simulink model "NM100A_MotVelCtrl"  (R2013b)
settings: Solver=FixedStepDiscrete  SolverMode=SingleTasking  StartTime=0.0  StopTime=1  FixedStep=0.002  RelTol=1e-3
values from neighbouring files (symbols this model uses):
  ARCHGLBPRM_2MILLISEC_SEC_F32 = DataDict.Constant    [NM100A_MotVelCtrl_DataDict.m]
  DERIVTVLPFILTICONLOWRLIM_SEC_F32 = DataDict.Constant    [NM100A_MotVelCtrl_DataDict.m]
  FALSE_CNT_LGC = DataDict.Constant    [NM100A_MotVelCtrl_DataDict.m]
  MOTVELTHDRAMPDWNCMPL_MOTRADPERSEC_F32 = DataDict.Constant    [NM100A_MotVelCtrl_DataDict.m]
  ONEMILLISEC_SEC_F32 = DataDict.Constant    [NM100A_MotVelCtrl_DataDict.m]
  TITHDRAMPDWNCMPL_CNT_U16 = DataDict.Constant    [NM100A_MotVelCtrl_DataDict.m]
  TRUE_CNT_LGC = DataDict.Constant    [NM100A_MotVelCtrl_DataDict.m]
  ZEROMOTVELTAR_MOTRADPERSEC_F32 = DataDict.Constant    [NM100A_MotVelCtrl_DataDict.m]
  ZEROTQCMD_MOTNWTMTR_F32 = DataDict.Constant    [NM100A_MotVelCtrl_DataDict.m]
libraries: NxtrLim x13, simulink x1, NxtrAbslt x1, NxtrMax x1
(part 1 of 4)
settings Model: Creator=DZVCQL  LastModifiedBy=DZVCQL
settings SolverCC: AutoInsertRateTranBlk=on  InsertRTBMode=Always
settings DataIOCC: LimitDataPoints=off  SaveFormat=Structure  ReturnWorkspaceOutputs=on
settings OptimizationCC: BlockReduction=off  InlineParams=on  ZeroExternalMemoryAtStartup=off  ZeroInternalMemoryAtStartup=off  OptimizeModelRefInitCode=on  LifeSpan=1
settings DebuggingCC: SignalInfNanChecking=error  SignalRangeChecking=warning  ReadBeforeWriteMsg=DisableAll  WriteAfterWriteMsg=DisableAll  WriteAfterReadMsg=DisableAll  UnderspecifiedInitializationDetection=Simplified  SolverPrmCheckMsg=error  InheritedTsInSrcMsg=error  DiscreteInheritContinuousMsg=error  SingleTaskRateTransMsg=error  TasksWithSamePriorityMsg=error  SigSpecEnsureSampleTimeMsg=error  CheckMatrixSingularityMsg=error  ParameterUnderflowMsg=error  ParameterPrecisionLossMsg=error  ParameterTunabilityLossMsg=error  FixptConstUnderflowMsg=warning  FixptConstOverflowMsg=warning  VectorMatrixConversionMsg=error  SignalLabelMismatchMsg=error  UnconnectedInputMsg=error  UnconnectedOutputMsg=error  UnconnectedLineMsg=error  SFcnCompatibilityMsg=error  UniqueDataStoreMsg=warning  BusObjectLabelMismatch=error  RootOutportRequireBusObject=error  AssertControl=DisableAll  ModelReferenceIOMsg=error  ModelReferenceVersionMismatchMessage=warning  ModelReferenceIOMismatchMessage=error  ModelReferenceCSMismatchMessage=warning  ModelReferenceDataLoggingMessage=error  StateNameClashWarn=warning  StrictBusMsg=ErrorOnBusTreatedAsVector  NonBusSignalsTreatedAsBus=error  SFUnexpectedBacktrackingDiag=error  SFInvalidInputDataAccessInChartInitDiag=error  SFNoUnconditionalDefaultTransitionDiag=error  SFTransitionOutsideNaturalParentDiag=error  SFUnconditionalTransitionShadowingDiag=error  SFUndirectedBroadcastEventsDiag=error
settings ModelReferenceCC: ModelReferenceNumInstancesAllowed=Single
settings RTWCC: SystemTargetFile=autosar.tlc  GenCodeOnly=on  TemplateMakefile=ert_default_tmf  Description=AUTOSAR  GenerateReport=on  ProcessScript=autosar_make_rtw_hook  LaunchReport=on
settings CodeAppCC: GenerateComments=off  IgnoreCustomStorageClasses=off  CustomSymbolStrType=$N$R$M  CustomSymbolStrBlkIO=$N$M  SimulinkBlockComments=off
settings STFCustomTargetCC: ParMdlRefBuildCompliant=on  CompOptLevelCompliant=on  IncludeMdlTerminateFcn=off  CombineOutputUpdateFcns=on  SuppressErrorStatus=on  ERTFirstTimeCompliant=on  ERTCustomFileBanners=on  SupportNonFinite=off  SupportComplex=off  SupportContinuousTime=off  SupportNonInlinedSFcns=off  MATLABClassNameForMDSCustomization=Simulink.SoftwareTarget.ERTCustomization  AutosarCompliant=on  GRTInterface=off  SystemTargetFile=autosar.tlc
settings ERTTargetCC: CodeReplacementLibrary=ANSI_C  ConcurrentExecutionCompliant=off  IncludeMdlTerminateFcn=off  SuppressErrorStatus=on  SupportNonFinite=off  SupportComplex=off  ModelStepFunctionPrototypeControlCompliant=off  CPPClassGenCompliant=off  AutosarCompliant=on  InlinedParameterPlacement=NonHierarchical  ERTCustomFileTemplate=example_file_process.tlc  EnableUserReplacementTypes=on

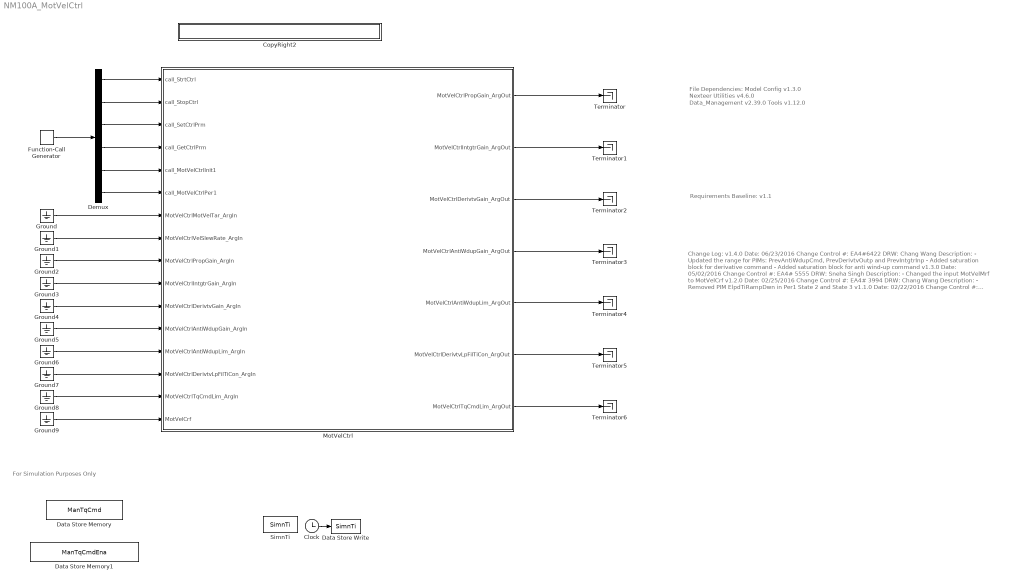
== system NM100A_MotVelCtrl ==
  note: Change Log:
      |
      | v1.4.0
      | Date: 06/23/2016
      | Change Control #: EA4#6422
      | DRW: Chang Wang
      | Description:
      | - Updated the range for PIMs: PrevAntiWdupCmd, PrevDerivtvOutp and PrevIntgtrInp
      | - Added saturation block for derivative command
      | - Added saturation block for anti wind-up command
      |
      | v1.3.0
      | Date: 05/02/2016
      | Change Control #: EA4# 5555
      | DRW: Sneha Singh
      | Description:
      | - Changed the input MotVelMrf to MotVelCrf
      |
      | v1.2.0
      | Date: 02/25/2016
      | Change Control #: EA4# 3994
      | DRW: Chang Wang
      | Description:
      | - Removed PIM ElpdTiRampDwn in Per1 State 2 and State 3
      |
      | v1.1.0
      | Date: 02/22/2016
      | Change Control #: EA4# 3954
      | DRW: Chang Wang
      | Description:
      | - Added client definition in data dictionary
      |
      | v1.0.0
      | Date: 02/09/2016
      | Change Control #: EA4# 2604
      | DRW: Chang Wang
      | Description:
      | - Initial Release
  note: Requirements Baseline: v1.1
  note: File Dependencies:
      |
      | Model Config v1.3.0
      | Nexteer Utilities v4.6.0
      | Data_Management v2.39.0
      | Tools v1.12.0
  note: For Simulation Purposes Only
  Clock : Clock
  CopyRight2 : Subsystem  Description=|  mask(Copyright Information){none=on}
      | Copyright info block.                                               
      |                                                                     
      | Place copyright information at the top of every subsystem in design.
      mask prompts: none "No parameters"
      mask help: Place copyright information at the top of every subsystem in design.
      mask Display:
      | NxtrConf = 'Nexteer Confidential';
      | 
      | sys = bdroot; %handle for the current model ("system")
      | first = get_param(sys,'Created');
      | if(isempty(first))
      |     first = datestr(now,'yyyy');
      | else
      |     first = first(end-3:end);  %year is last four digits
      | end
      | 
      | last = get_param(sys,'LastModifiedDate');
      | if isempty(last)
      |     last = datestr(now,'yyyy');
      | else
      |     last = last(end-3:end);
      | end
      | 
      | if strcmp(first,last)
      |     fprintf('%s -- Copyright %s Nexteer',NxtrConf,first)
      | else
      |     fprintf('%s -- %s%s- %s Nexteer',NxtrConf,char(169),first,last)
      | end
  Data Store Memory : DataStoreMemory  DataStoreName=ManTqCmd  ReadBeforeWriteMsg=warning  WriteAfterWriteMsg=warning  WriteAfterReadMsg=warning
  Data Store Memory1 : DataStoreMemory  DataStoreName=ManTqCmdEna  ReadBeforeWriteMsg=warning  WriteAfterWriteMsg=warning  WriteAfterReadMsg=warning
  Data Store Write : DataStoreWrite  DataStoreName=SimnTi
  Demux : Demux  Outputs=6
  Function-Call Generator : simulink/Ports & Subsystems/Function-Call Generator  sample_time=0.002  numberOfIterations=1
  Ground{,1..8} (9 alike) : Ground
  Ground9 : Ground  RequirementInfo="{}  %GIDa_4af75635_9092_474e_b30d_2604ca9b8832"
  MotVelCtrl : Subsystem
  SimnTi : DataStoreMemory  DataStoreName=SimnTi
  Terminator{,1..6} (7 alike) : Terminator
  wires:
  Demux/1 -> MotVelCtrl/1(call_StrtCtrl)
  Demux/2 -> MotVelCtrl/2(call_StopCtrl)
  Demux/3 -> MotVelCtrl/3(call_SetCtrlPrm)
  Demux/4 -> MotVelCtrl/4(call_GetCtrlPrm)
  Demux/5 -> MotVelCtrl/5(call_MotVelCtrlInit1)
  Demux/6 -> MotVelCtrl/6(call_MotVelCtrlPer1)
  Function-Call Generator/1 -> Demux/1
  Ground9/1 -> MotVelCtrl/16(MotVelCrf)
  Ground8/1 -> MotVelCtrl/15(MotVelCtrlTqCmdLim_ArgIn)
  Ground7/1 -> MotVelCtrl/14(MotVelCtrlDerivtvLpFilTiCon_ArgIn)
  Ground6/1 -> MotVelCtrl/13(MotVelCtrlAntiWdupLim_ArgIn)
  Ground5/1 -> MotVelCtrl/12(MotVelCtrlAntiWdupGain_ArgIn)
  Ground4/1 -> MotVelCtrl/11(MotVelCtrlDerivtvGain_ArgIn)
  Ground3/1 -> MotVelCtrl/10(MotVelCtrlIntgtrGain_ArgIn)
  Ground2/1 -> MotVelCtrl/9(MotVelCtrlPropGain_ArgIn)
  Ground1/1 -> MotVelCtrl/8(MotVelCtrlVelSlewRate_ArgIn)
  Ground/1 -> MotVelCtrl/7(MotVelCtrlMotVelTar_ArgIn)
  MotVelCtrl/1(MotVelCtrlPropGain_ArgOut) -> Terminator/1
  MotVelCtrl/2(MotVelCtrlIntgtrGain_ArgOut) -> Terminator1/1
  MotVelCtrl/3(MotVelCtrlDerivtvGain_ArgOut) -> Terminator2/1
  MotVelCtrl/4(MotVelCtrlAntiWdupGain_ArgOut) -> Terminator3/1
  MotVelCtrl/5(MotVelCtrlAntiWdupLim_ArgOut) -> Terminator4/1
  MotVelCtrl/6(MotVelCtrlDerivtvLpFilTiCon_ArgOut) -> Terminator5/1
  MotVelCtrl/7(MotVelCtrlTqCmdLim_ArgOut) -> Terminator6/1
  Clock/1 -> Data Store Write/1

== system NM100A_MotVelCtrl/CopyRight2 ==

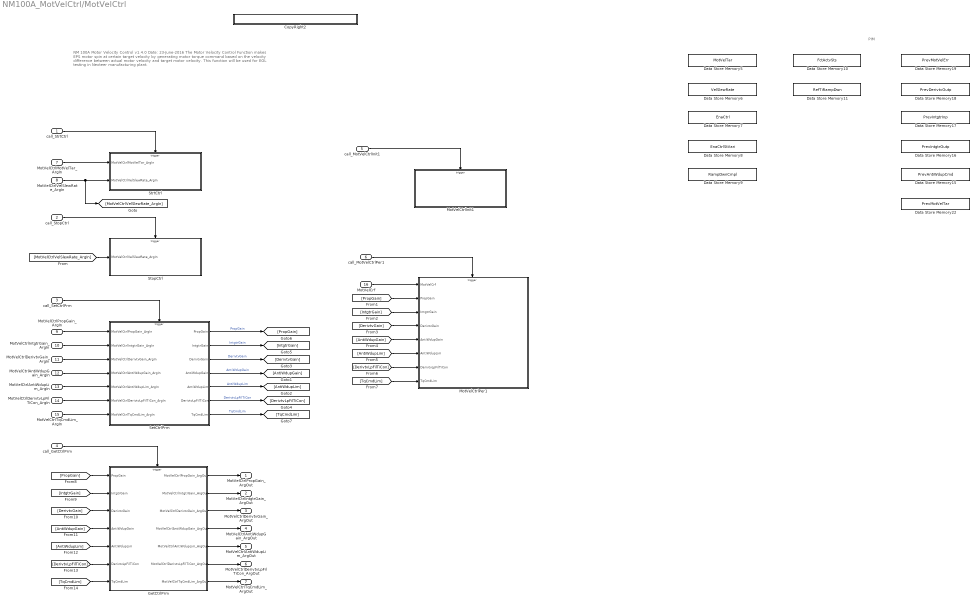
== system NM100A_MotVelCtrl/MotVelCtrl ==
  note: PIM
  note: NM 100A  Motor Velocity Control
      | v1.4.0      Date: 23-June-2016
      |
      | The Motor Velocity Control Function makes EPS motor spin at certain target velocity by generating motor torque command based on the
      | velocity difference between actual motor velocity and target motor velocity. This function will be used for EOL testing in Nexteer manufacturing
      | plant.
  call_StrtCtrl : Inport
  call_StopCtrl : Inport  Port=2
  call_SetCtrlPrm : Inport  Port=3
  call_GetCtrlPrm : Inport  Port=4
  call_MotVelCtrlInit1 : Inport  Port=5
  call_MotVelCtrlPer1 : Inport  Port=6
  MotVelCtrlMotVelTar_ArgIn : Inport  RequirementInfo="{'linktype_rmi_doors' '00010020 (/E-STEER Core/SubSystem Specifications/Manufacturing Service/NM100A_Motor Velocity Control Function Requirement)' '#NM100A_10' 'true' 'REQ:  NM100A_10' '' ; 'linktype_rmi_doors' '00010020 (/E-STEER Core/SubSystem Specifications/Manufacturing Service/NM100A_Motor Velocity Control Function Requirement)' '#NM100A_84' 'true' 'REQ:  NM100A_84' '' } %GIDa_b4e5afd2_56f5_46d2_aa0a_1f9c462eceac"  Port=7
  MotVelCtrlVelSlewRate_ArgIn : Inport  RequirementInfo="{'linktype_rmi_doors' '00010020 (/E-STEER Core/SubSystem Specifications/Manufacturing Service/NM100A_Motor Velocity Control Function Requirement)' '#NM100A_11' 'true' 'REQ:  NM100A_11' '' ; 'linktype_rmi_doors' '00010020 (/E-STEER Core/SubSystem Specifications/Manufacturing Service/NM100A_Motor Velocity Control Function Requirement)' '#NM100A_84' 'true' 'REQ:  NM100A_84' '' } %GIDa_6a002315_8dfa_4d7e_b831_7383949bc30b"  Port=8
  MotVelCtrlPropGain_ArgIn : Inport  RequirementInfo="{'linktype_rmi_doors' '00010020 (/E-STEER Core/SubSystem Specifications/Manufacturing Service/NM100A_Motor Velocity Control Function Requirement)' '#NM100A_13' 'true' 'REQ:  NM100A_13' '' ; 'linktype_rmi_doors' '00010020 (/E-STEER Core/SubSystem Specifications/Manufacturing Service/NM100A_Motor Velocity Control Function Requirement)' '#NM100A_85' 'true' 'REQ:  NM100A_85' '' } %GIDa_fa7a9d38_ec4e_42af_8ef7_a516fd31c72a"  Port=9
  MotVelCtrlIntgtrGain_ArgIn : Inport  RequirementInfo="{'linktype_rmi_doors' '00010020 (/E-STEER Core/SubSystem Specifications/Manufacturing Service/NM100A_Motor Velocity Control Function Requirement)' '#NM100A_13' 'true' 'REQ:  NM100A_13' '' ; 'linktype_rmi_doors' '00010020 (/E-STEER Core/SubSystem Specifications/Manufacturing Service/NM100A_Motor Velocity Control Function Requirement)' '#NM100A_85' 'true' 'REQ:  NM100A_85' '' } %GIDa_da1bc328_85e1_4524_82bb_c455a15a83f5"  Port=10
  MotVelCtrlDerivtvGain_ArgIn : Inport  RequirementInfo="{'linktype_rmi_doors' '00010020 (/E-STEER Core/SubSystem Specifications/Manufacturing Service/NM100A_Motor Velocity Control Function Requirement)' '#NM100A_13' 'true' 'REQ:  NM100A_13' '' ; 'linktype_rmi_doors' '00010020 (/E-STEER Core/SubSystem Specifications/Manufacturing Service/NM100A_Motor Velocity Control Function Requirement)' '#NM100A_85' 'true' 'REQ:  NM100A_85' '' } %GIDa_c5db38f5_dbd5_422b_8505_a0e67da4c1c3"  Port=11
  MotVelCtrlAntiWdupGain_ArgIn : Inport  RequirementInfo="{'linktype_rmi_doors' '00010020 (/E-STEER Core/SubSystem Specifications/Manufacturing Service/NM100A_Motor Velocity Control Function Requirement)' '#NM100A_14' 'true' 'REQ:  NM100A_14' '' ; 'linktype_rmi_doors' '00010020 (/E-STEER Core/SubSystem Specifications/Manufacturing Service/NM100A_Motor Velocity Control Function Requirement)' '#NM100A_85' 'true' 'REQ:  NM100A_85' '' } %GIDa_dd319c0c_aa78_494d_974e_a4fd1e8fae44"  Port=12
  MotVelCtrlAntiWdupLim_ArgIn : Inport  RequirementInfo="{'linktype_rmi_doors' '00010020 (/E-STEER Core/SubSystem Specifications/Manufacturing Service/NM100A_Motor Velocity Control Function Requirement)' '#NM100A_14' 'true' 'REQ:  NM100A_14' '' ; 'linktype_rmi_doors' '00010020 (/E-STEER Core/SubSystem Specifications/Manufacturing Service/NM100A_Motor Velocity Control Function Requirement)' '#NM100A_85' 'true' 'REQ:  NM100A_85' '' } %GIDa_0e3b6542_1c91_470d_a92d_ce3c261459b8"  Port=13
  MotVelCtrlDerivtvLpFilTiCon_ArgIn : Inport  RequirementInfo="{'linktype_rmi_doors' '00010020 (/E-STEER Core/SubSystem Specifications/Manufacturing Service/NM100A_Motor Velocity Control Function Requirement)' '#NM100A_15' 'true' 'REQ:  NM100A_15' '' ; 'linktype_rmi_doors' '00010020 (/E-STEER Core/SubSystem Specifications/Manufacturing Service/NM100A_Motor Velocity Control Function Requirement)' '#NM100A_85' 'true' 'REQ:  NM100A_85' '' } %GIDa_cfe3ce5c_c322_4f86_b6db_5a668332a15c"  Port=14
  MotVelCtrlTqCmdLim_ArgIn : Inport  RequirementInfo="{'linktype_rmi_doors' '00010020 (/E-STEER Core/SubSystem Specifications/Manufacturing Service/NM100A_Motor Velocity Control Function Requirement)' '#NM100A_16' 'true' 'REQ:  NM100A_16' '' ; 'linktype_rmi_doors' '00010020 (/E-STEER Core/SubSystem Specifications/Manufacturing Service/NM100A_Motor Velocity Control Function Requirement)' '#NM100A_85' 'true' 'REQ:  NM100A_85' '' } %GIDa_2c1dfec7_b849_4afb_8c15_4e0ef5eb7c29"  Port=15
  MotVelCrf : Inport  RequirementInfo="{'linktype_rmi_doors' '00010020 (/E-STEER Core/SubSystem Specifications/Manufacturing Service/NM100A_Motor Velocity Control Function Requirement)' '#NM100A_9' 'true' 'REQ:  NM100A_9' '' } %GIDa_78fb18dd_9313_48f8_8b5a_3efff0ddc69b"  Port=16
  CopyRight2 : Subsystem  Description=|  mask(Copyright Information){none=on}
      | Copyright info block.                                               
      |                                                                     
      | Place copyright information at the top of every subsystem in design.
      mask prompts: none "No parameters"
      mask help: Place copyright information at the top of every subsystem in design.
      mask Display:
      | NxtrConf = 'Nexteer Confidential';
      | 
      | sys = bdroot; %handle for the current model ("system")
      | first = get_param(sys,'Created');
      | if(isempty(first))
      |     first = datestr(now,'yyyy');
      | else
      |     first = first(end-3:end);  %year is last four digits
      | end
      | 
      | last = get_param(sys,'LastModifiedDate');
      | if isempty(last)
      |     last = datestr(now,'yyyy');
      | else
      |     last = last(end-3:end);
      | end
      | 
      | if strcmp(first,last)
      |     fprintf('%s -- Copyright %s Nexteer',NxtrConf,first)
      | else
      |     fprintf('%s -- %s%s- %s Nexteer',NxtrConf,char(169),first,last)
      | end
  Data Store Memory10 : DataStoreMemory  DataStoreName=FctActvSts  ReadBeforeWriteMsg=warning  WriteAfterWriteMsg=warning  WriteAfterReadMsg=warning  StateMustResolveToSignalObject=on
  Data Store Memory11 : DataStoreMemory  DataStoreName=RefTiRampDwn  ReadBeforeWriteMsg=warning  WriteAfterWriteMsg=warning  WriteAfterReadMsg=warning  StateMustResolveToSignalObject=on
  Data Store Memory15 : DataStoreMemory  DataStoreName=PrevAntiWdupCmd  ReadBeforeWriteMsg=warning  WriteAfterWriteMsg=warning  WriteAfterReadMsg=warning  StateMustResolveToSignalObject=on
  Data Store Memory16 : DataStoreMemory  DataStoreName=PrevIntgtrOutp  ReadBeforeWriteMsg=warning  WriteAfterWriteMsg=warning  WriteAfterReadMsg=warning  StateMustResolveToSignalObject=on
  Data Store Memory17 : DataStoreMemory  DataStoreName=PrevIntgtrInp  ReadBeforeWriteMsg=warning  WriteAfterWriteMsg=warning  WriteAfterReadMsg=warning  StateMustResolveToSignalObject=on
  Data Store Memory18 : DataStoreMemory  DataStoreName=PrevDerivtvOutp  ReadBeforeWriteMsg=warning  WriteAfterWriteMsg=warning  WriteAfterReadMsg=warning  StateMustResolveToSignalObject=on
  Data Store Memory19 : DataStoreMemory  DataStoreName=PrevMotVelErr  ReadBeforeWriteMsg=warning  WriteAfterWriteMsg=warning  WriteAfterReadMsg=warning  StateMustResolveToSignalObject=on
  Data Store Memory22 : DataStoreMemory  DataStoreName=PrevMotVelTar  ReadBeforeWriteMsg=warning  WriteAfterWriteMsg=warning  WriteAfterReadMsg=warning  StateMustResolveToSignalObject=on
  Data Store Memory5 : DataStoreMemory  DataStoreName=MotVelTar  ReadBeforeWriteMsg=warning  WriteAfterWriteMsg=warning  WriteAfterReadMsg=warning  StateMustResolveToSignalObject=on
  Data Store Memory6 : DataStoreMemory  DataStoreName=VelSlewRate  ReadBeforeWriteMsg=warning  WriteAfterWriteMsg=warning  WriteAfterReadMsg=warning  StateMustResolveToSignalObject=on
  Data Store Memory7 : DataStoreMemory  DataStoreName=EnaCtrl  ReadBeforeWriteMsg=warning  WriteAfterWriteMsg=warning  WriteAfterReadMsg=warning  StateMustResolveToSignalObject=on
  Data Store Memory8 : DataStoreMemory  DataStoreName=EnaCtrlStVari  ReadBeforeWriteMsg=warning  WriteAfterWriteMsg=warning  WriteAfterReadMsg=warning  StateMustResolveToSignalObject=on
  Data Store Memory9 : DataStoreMemory  DataStoreName=RampDwnCmpl  ReadBeforeWriteMsg=warning  WriteAfterWriteMsg=warning  WriteAfterReadMsg=warning  StateMustResolveToSignalObject=on
  GetCtrlPrm : Subsystem  TreatAsAtomicUnit=on
  MotVelCtrlInit1 : Subsystem  TreatAsAtomicUnit=on
  MotVelCtrlPer1 : Subsystem  TreatAsAtomicUnit=on
  SetCtrlPrm : Subsystem  TreatAsAtomicUnit=on
  StopCtrl : Subsystem  TreatAsAtomicUnit=on
  StrtCtrl : Subsystem  TreatAsAtomicUnit=on
  MotVelCtrlPropGain_ArgOut : Outport  RequirementInfo="{'linktype_rmi_doors' '00010020 (/E-STEER Core/SubSystem Specifications/Manufacturing Service/NM100A_Motor Velocity Control Function Requirement)' '#NM100A_105' 'true' 'REQ:  NM100A_105' '' ; 'linktype_rmi_doors' '00010020 (/E-STEER Core/SubSystem Specifications/Manufacturing Service/NM100A_Motor Velocity Control Function Requirement)' '#NM100A_86' 'true' 'REQ:  NM100A_86' '' } %GIDa_fbcf257f_3a7e_4784_95d9_7f44ee96f49e"
  MotVelCtrlIntgtrGain_ArgOut : Outport  RequirementInfo="{'linktype_rmi_doors' '00010020 (/E-STEER Core/SubSystem Specifications/Manufacturing Service/NM100A_Motor Velocity Control Function Requirement)' '#NM100A_105' 'true' 'REQ:  NM100A_105' '' ; 'linktype_rmi_doors' '00010020 (/E-STEER Core/SubSystem Specifications/Manufacturing Service/NM100A_Motor Velocity Control Function Requirement)' '#NM100A_86' 'true' 'REQ:  NM100A_86' '' } %GIDa_a30212a1_db40_493f_99ad_7cd60670be6b"  Port=2
  MotVelCtrlDerivtvGain_ArgOut : Outport  RequirementInfo="{'linktype_rmi_doors' '00010020 (/E-STEER Core/SubSystem Specifications/Manufacturing Service/NM100A_Motor Velocity Control Function Requirement)' '#NM100A_105' 'true' 'REQ:  NM100A_105' '' ; 'linktype_rmi_doors' '00010020 (/E-STEER Core/SubSystem Specifications/Manufacturing Service/NM100A_Motor Velocity Control Function Requirement)' '#NM100A_86' 'true' 'REQ:  NM100A_86' '' } %GIDa_d511169f_960f_4b26_aa3f_53333eb486bd"  Port=3
  MotVelCtrlAntiWdupGain_ArgOut : Outport  RequirementInfo="{'linktype_rmi_doors' '00010020 (/E-STEER Core/SubSystem Specifications/Manufacturing Service/NM100A_Motor Velocity Control Function Requirement)' '#NM100A_107' 'true' 'REQ:  NM100A_107' '' ; 'linktype_rmi_doors' '00010020 (/E-STEER Core/SubSystem Specifications/Manufacturing Service/NM100A_Motor Velocity Control Function Requirement)' '#NM100A_86' 'true' 'REQ:  NM100A_86' '' } %GIDa_da526535_3849_41c7_869e_59d948236c9d"  Port=4
  MotVelCtrlAntiWdupLim_ArgOut : Outport  RequirementInfo="{'linktype_rmi_doors' '00010020 (/E-STEER Core/SubSystem Specifications/Manufacturing Service/NM100A_Motor Velocity Control Function Requirement)' '#NM100A_107' 'true' 'REQ:  NM100A_107' '' ; 'linktype_rmi_doors' '00010020 (/E-STEER Core/SubSystem Specifications/Manufacturing Service/NM100A_Motor Velocity Control Function Requirement)' '#NM100A_86' 'true' 'REQ:  NM100A_86' '' } %GIDa_a2928b64_1a88_4f0b_886a_22a0a7f92bff"  Port=5
  MotVelCtrlDerivtvLpFilTiCon_ArgOut : Outport  RequirementInfo="{'linktype_rmi_doors' '00010020 (/E-STEER Core/SubSystem Specifications/Manufacturing Service/NM100A_Motor Velocity Control Function Requirement)' '#NM100A_108' 'true' 'REQ:  NM100A_108' '' ; 'linktype_rmi_doors' '00010020 (/E-STEER Core/SubSystem Specifications/Manufacturing Service/NM100A_Motor Velocity Control Function Requirement)' '#NM100A_86' 'true' 'REQ:  NM100A_86' '' } %GIDa_e78ab4ff_8646_49da_9642_5dd7cce604f1"  Port=6
  MotVelCtrlTqCmdLim_ArgOut : Outport  RequirementInfo="{'linktype_rmi_doors' '00010020 (/E-STEER Core/SubSystem Specifications/Manufacturing Service/NM100A_Motor Velocity Control Function Requirement)' '#NM100A_109' 'true' 'REQ:  NM100A_109' '' ; 'linktype_rmi_doors' '00010020 (/E-STEER Core/SubSystem Specifications/Manufacturing Service/NM100A_Motor Velocity Control Function Requirement)' '#NM100A_86' 'true' 'REQ:  NM100A_86' '' } %GIDa_332bdf64_fdb5_47d8_90a4_34844676e793"  Port=7
  wires:
  call_StrtCtrl/1 -> StrtCtrl/Trigger
  MotVelCtrlMotVelTar_ArgIn/1 -> StrtCtrl/1(MotVelCtrlMotVelTar_ArgIn)
  MotVelCtrlVelSlewRate_ArgIn/1 -> [MotVelCtrlVelSlewRate_ArgIn], StrtCtrl/2(MotVelCtrlVelSlewRate_ArgIn)
  call_StopCtrl/1 -> StopCtrl/Trigger
  call_SetCtrlPrm/1 -> SetCtrlPrm/Trigger
  MotVelCtrlPropGain_ArgIn/1 -> SetCtrlPrm/1(MotVelCtrlPropGain_ArgIn)
  MotVelCtrlIntgtrGain_ArgIn/1 -> SetCtrlPrm/2(MotVelCtrlIntgtrGain_ArgIn)
  MotVelCtrlDerivtvGain_ArgIn/1 -> SetCtrlPrm/3(MotVelCtrlDerivtvGain_ArgIn)
  call_GetCtrlPrm/1 -> GetCtrlPrm/Trigger
  MotVelCtrlAntiWdupGain_ArgIn/1 -> SetCtrlPrm/4(MotVelCtrlAntiWdupGain_ArgIn)
  MotVelCtrlAntiWdupLim_ArgIn/1 -> SetCtrlPrm/5(MotVelCtrlAntiWdupLim_ArgIn)
  MotVelCtrlDerivtvLpFilTiCon_ArgIn/1 -> SetCtrlPrm/6(MotVelCtrlDerivtvLpFilTiCon_ArgIn)
  MotVelCtrlTqCmdLim_ArgIn/1 -> SetCtrlPrm/7(MotVelCtrlTqCmdLim_ArgIn)
  GetCtrlPrm/1(MotVelCtrlPropGain_ArgOut) -> MotVelCtrlPropGain_ArgOut/1
  GetCtrlPrm/2(MotVelCtrlIntgtrGain_ArgOut) -> MotVelCtrlIntgtrGain_ArgOut/1
  GetCtrlPrm/7(MotVelCtrlTqCmdLim_ArgOut) -> MotVelCtrlTqCmdLim_ArgOut/1
  GetCtrlPrm/6(MotVelCtrlDerivtvLpFilTiCon_ArgOut) -> MotVelCtrlDerivtvLpFilTiCon_ArgOut/1
  GetCtrlPrm/5(MotVelCtrlAntiWdupLim_ArgOut) -> MotVelCtrlAntiWdupLim_ArgOut/1
  GetCtrlPrm/4(MotVelCtrlAntiWdupGain_ArgOut) -> MotVelCtrlAntiWdupGain_ArgOut/1
  GetCtrlPrm/3(MotVelCtrlDerivtvGain_ArgOut) -> MotVelCtrlDerivtvGain_ArgOut/1
  [MotVelCtrlVelSlewRate_ArgIn] -> StopCtrl/1(MotVelCtrlVelSlewRate_ArgIn)
  call_MotVelCtrlPer1/1 -> MotVelCtrlPer1/Trigger
  MotVelCrf/1 -> MotVelCtrlPer1/1(MotVelCrf)
  call_MotVelCtrlInit1/1 -> MotVelCtrlInit1/Trigger
  SetCtrlPrm/1(PropGain) -> [PropGain]  "PropGain"
  SetCtrlPrm/2(IntgtrGain) -> [IntgtrGain]  "IntgtrGain"
  SetCtrlPrm/3(DerivtvGain) -> [DerivtvGain]  "DerivtvGain"
  SetCtrlPrm/4(AntiWdupGain) -> [AntiWdupGain]  "AntiWdupGain"
  SetCtrlPrm/5(AntiWdupLim) -> [AntiWdupLim]  "AntiWdupLim"
  SetCtrlPrm/6(DerivtvLpFilTiCon) -> [DerivtvLpFilTiCon]  "DerivtvLpFilTiCon"
  SetCtrlPrm/7(TqCmdLim) -> [TqCmdLim]  "TqCmdLim"
  [PropGain] -> GetCtrlPrm/1(PropGain)
  [IntgtrGain] -> GetCtrlPrm/2(IntgtrGain)
  [DerivtvGain] -> GetCtrlPrm/3(DerivtvGain)
  [AntiWdupGain] -> GetCtrlPrm/4(AntiWdupGain)
  [AntiWdupLim] -> GetCtrlPrm/5(AntiWdupLim)
  [DerivtvLpFilTiCon] -> GetCtrlPrm/6(DerivtvLpFilTiCon)
  [TqCmdLim] -> GetCtrlPrm/7(TqCmdLim)
  [PropGain] -> MotVelCtrlPer1/2(PropGain)
  [IntgtrGain] -> MotVelCtrlPer1/3(IntgtrGain)
  [DerivtvGain] -> MotVelCtrlPer1/4(DerivtvGain)
  [AntiWdupGain] -> MotVelCtrlPer1/5(AntiWdupGain)
  [AntiWdupLim] -> MotVelCtrlPer1/6(AntiWdupLim)
  [DerivtvLpFilTiCon] -> MotVelCtrlPer1/7(DerivtvLpFilTiCon)
  [TqCmdLim] -> MotVelCtrlPer1/8(TqCmdLim)

== system NM100A_MotVelCtrl/MotVelCtrl/CopyRight2 ==

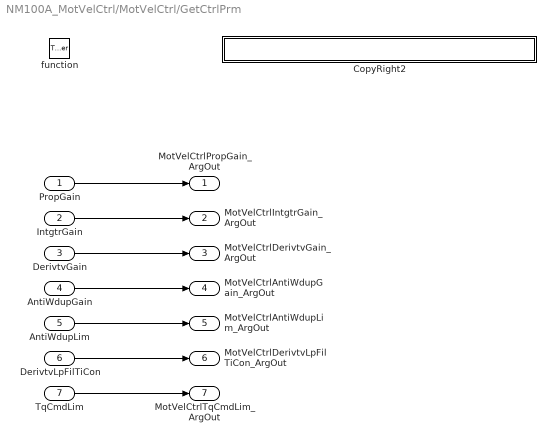
== system NM100A_MotVelCtrl/MotVelCtrl/GetCtrlPrm ==
  PropGain : Inport
  IntgtrGain : Inport  Port=2
  DerivtvGain : Inport  Port=3
  AntiWdupGain : Inport  Port=4
  AntiWdupLim : Inport  Port=5
  DerivtvLpFilTiCon : Inport  Port=6
  TqCmdLim : Inport  Port=7
  function : TriggerPort  TriggerType=function-call
  CopyRight2 : Subsystem  Description=|  mask(Copyright Information){none=on}
      | Copyright info block.                                               
      |                                                                     
      | Place copyright information at the top of every subsystem in design.
      mask prompts: none "No parameters"
      mask help: Place copyright information at the top of every subsystem in design.
      mask Display:
      | NxtrConf = 'Nexteer Confidential';
      | 
      | sys = bdroot; %handle for the current model ("system")
      | first = get_param(sys,'Created');
      | if(isempty(first))
      |     first = datestr(now,'yyyy');
      | else
      |     first = first(end-3:end);  %year is last four digits
      | end
      | 
      | last = get_param(sys,'LastModifiedDate');
      | if isempty(last)
      |     last = datestr(now,'yyyy');
      | else
      |     last = last(end-3:end);
      | end
      | 
      | if strcmp(first,last)
      |     fprintf('%s -- Copyright %s Nexteer',NxtrConf,first)
      | else
      |     fprintf('%s -- %s%s- %s Nexteer',NxtrConf,char(169),first,last)
      | end
  MotVelCtrlPropGain_ArgOut : Outport
  MotVelCtrlIntgtrGain_ArgOut : Outport  Port=2
  MotVelCtrlDerivtvGain_ArgOut : Outport  Port=3
  MotVelCtrlAntiWdupGain_ArgOut : Outport  Port=4
  MotVelCtrlAntiWdupLim_ArgOut : Outport  Port=5
  MotVelCtrlDerivtvLpFilTiCon_ArgOut : Outport  Port=6
  MotVelCtrlTqCmdLim_ArgOut : Outport  Port=7
  wires:
  TqCmdLim/1 -> MotVelCtrlTqCmdLim_ArgOut/1
  DerivtvLpFilTiCon/1 -> MotVelCtrlDerivtvLpFilTiCon_ArgOut/1
  AntiWdupLim/1 -> MotVelCtrlAntiWdupLim_ArgOut/1
  AntiWdupGain/1 -> MotVelCtrlAntiWdupGain_ArgOut/1
  DerivtvGain/1 -> MotVelCtrlDerivtvGain_ArgOut/1
  IntgtrGain/1 -> MotVelCtrlIntgtrGain_ArgOut/1
  PropGain/1 -> MotVelCtrlPropGain_ArgOut/1

== system NM100A_MotVelCtrl/MotVelCtrl/MotVelCtrlInit1 ==
  function : TriggerPort  TriggerType=function-call
  Constant : Constant  Value=FALSE_CNT_LGC
  Constant1 : Constant  Value=FALSE_CNT_LGC
  Constant2 : Constant  Value=TRUE_CNT_LGC
  Constant3 : Constant  Value=FALSE_CNT_LGC
  CopyRight2 : Subsystem  Description=|  mask(Copyright Information){none=on}
      | Copyright info block.                                               
      |                                                                     
      | Place copyright information at the top of every subsystem in design.
      mask prompts: none "No parameters"
      mask help: Place copyright information at the top of every subsystem in design.
      mask Display:
      | NxtrConf = 'Nexteer Confidential';
      | 
      | sys = bdroot; %handle for the current model ("system")
      | first = get_param(sys,'Created');
      | if(isempty(first))
      |     first = datestr(now,'yyyy');
      | else
      |     first = first(end-3:end);  %year is last four digits
      | end
      | 
      | last = get_param(sys,'LastModifiedDate');
      | if isempty(last)
      |     last = datestr(now,'yyyy');
      | else
      |     last = last(end-3:end);
      | end
      | 
      | if strcmp(first,last)
      |     fprintf('%s -- Copyright %s Nexteer',NxtrConf,first)
      | else
      |     fprintf('%s -- %s%s- %s Nexteer',NxtrConf,char(169),first,last)
      | end
  Data Store Write : DataStoreWrite  DataStoreName=EnaCtrl
  Data Store Write1 : DataStoreWrite  DataStoreName=EnaCtrlStVari
  Data Store Write2 : DataStoreWrite  DataStoreName=RampDwnCmpl
  Data Store Write3 : DataStoreWrite  DataStoreName=FctActvSts
  wires:
  Constant/1 -> Data Store Write/1
  Constant1/1 -> Data Store Write1/1
  Constant2/1 -> Data Store Write2/1
  Constant3/1 -> Data Store Write3/1

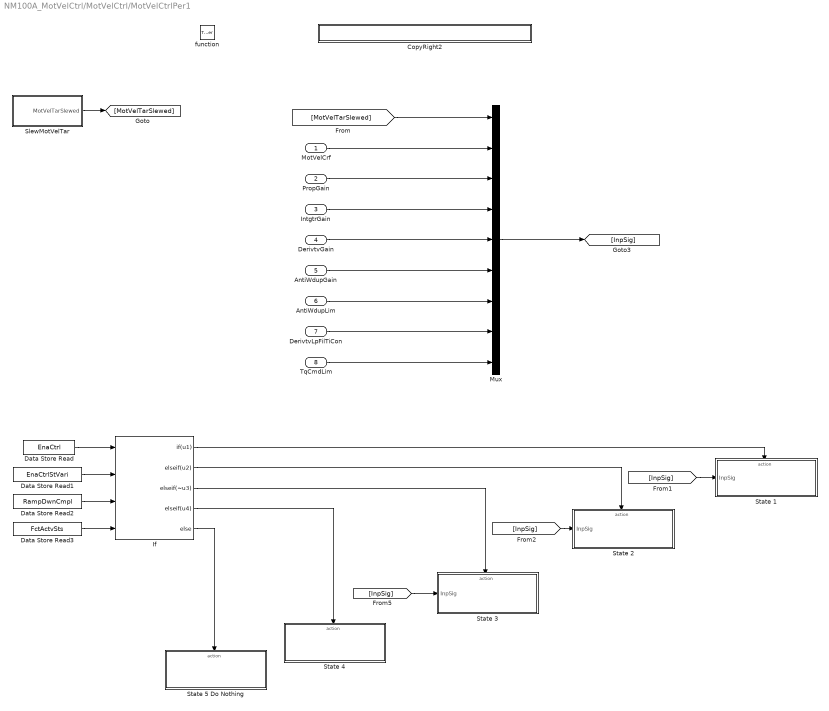
== system NM100A_MotVelCtrl/MotVelCtrl/MotVelCtrlPer1 ==
  MotVelCrf : Inport  RequirementInfo={} %GIDa_f6b199e4_d761_4852_9315_a0e807dc48bc
  PropGain : Inport  Port=2
  IntgtrGain : Inport  Port=3
  DerivtvGain : Inport  Port=4
  AntiWdupGain : Inport  Port=5
  AntiWdupLim : Inport  Port=6
  DerivtvLpFilTiCon : Inport  Port=7
  TqCmdLim : Inport  Port=8
  function : TriggerPort  TriggerType=function-call
  CopyRight2 : Subsystem  Description=|  mask(Copyright Information){none=on}
      | Copyright info block.                                               
      |                                                                     
      | Place copyright information at the top of every subsystem in design.
      mask prompts: none "No parameters"
      mask help: Place copyright information at the top of every subsystem in design.
      mask Display:
      | NxtrConf = 'Nexteer Confidential';
      | 
      | sys = bdroot; %handle for the current model ("system")
      | first = get_param(sys,'Created');
      | if(isempty(first))
      |     first = datestr(now,'yyyy');
      | else
      |     first = first(end-3:end);  %year is last four digits
      | end
      | 
      | last = get_param(sys,'LastModifiedDate');
      | if isempty(last)
      |     last = datestr(now,'yyyy');
      | else
      |     last = last(end-3:end);
      | end
      | 
      | if strcmp(first,last)
      |     fprintf('%s -- Copyright %s Nexteer',NxtrConf,first)
      | else
      |     fprintf('%s -- %s%s- %s Nexteer',NxtrConf,char(169),first,last)
      | end
  Data Store Read : DataStoreRead  RequirementInfo="{'linktype_rmi_doors' '00010020 (/E-STEER Core/SubSystem Specifications/Manufacturing Service/NM100A_Motor Velocity Control Function Requirement)' '#NM100A_48' 'true' 'REQ:  NM100A_48' '' ; 'linktype_rmi_doors' '00010020 (/E-STEER Core/SubSystem Specifications/Manufacturing Service/NM100A_Motor Velocity Control Function Requirement)' '#NM100A_49' 'true' 'REQ:  NM100A_49' '' ; 'linktype_rmi_doors' '00010020 (/E-STEER Core/SubSystem Specifications/Manufacturing Service/NM100A_Motor Velocity Control Function Requirement)' '#NM100A_51' 'true' 'REQ:  NM100A_51' '' ; 'linktype_rmi_doors' '00010020 (/E-STEER Core/SubSystem Specifications/Manufacturing Service/NM100A_Motor Velocity Control Function Requirement)' '#NM100A_103' 'true' 'REQ:  NM100A_103' '' } %GIDa_43add5bf_a7cd_4f8a_9e70_c6a4259d43f2"  DataStoreName=EnaCtrl
  Data Store Read1 : DataStoreRead  RequirementInfo="{'linktype_rmi_doors' '00010020 (/E-STEER Core/SubSystem Specifications/Manufacturing Service/NM100A_Motor Velocity Control Function Requirement)' '#NM100A_49' 'true' 'REQ:  NM100A_49' '' ; 'linktype_rmi_doors' '00010020 (/E-STEER Core/SubSystem Specifications/Manufacturing Service/NM100A_Motor Velocity Control Function Requirement)' '#NM100A_51' 'true' 'REQ:  NM100A_51' '' ; 'linktype_rmi_doors' '00010020 (/E-STEER Core/SubSystem Specifications/Manufacturing Service/NM100A_Motor Velocity Control Function Requirement)' '#NM100A_103' 'true' 'REQ:  NM100A_103' '' } %GIDa_56e92a46_fc14_4f42_a1bf_376f15bd98ae"  DataStoreName=EnaCtrlStVari
  Data Store Read2 : DataStoreRead  RequirementInfo="{'linktype_rmi_doors' '00010020 (/E-STEER Core/SubSystem Specifications/Manufacturing Service/NM100A_Motor Velocity Control Function Requirement)' '#NM100A_51' 'true' 'REQ:  NM100A_51' '' ; 'linktype_rmi_doors' '00010020 (/E-STEER Core/SubSystem Specifications/Manufacturing Service/NM100A_Motor Velocity Control Function Requirement)' '#NM100A_103' 'true' 'REQ:  NM100A_103' '' } %GIDa_d16d24dc_3caf_4308_b6b9_14741c0660fb"  DataStoreName=RampDwnCmpl
  Data Store Read3 : DataStoreRead  RequirementInfo="{'linktype_rmi_doors' '00010020 (/E-STEER Core/SubSystem Specifications/Manufacturing Service/NM100A_Motor Velocity Control Function Requirement)' '#NM100A_103' 'true' 'REQ:  NM100A_103' '' } %GIDa_dc81bd03_ef6f_4e75_8bbb_45c102c73405"  DataStoreName=FctActvSts
  If : If  RequirementInfo="{'linktype_rmi_doors' '00010020 (/E-STEER Core/SubSystem Specifications/Manufacturing Service/NM100A_Motor Velocity Control Function Requirement)' '#NM100A_48' 'true' 'REQ:  NM100A_48' '' ; 'linktype_rmi_doors' '00010020 (/E-STEER Core/SubSystem Specifications/Manufacturing Service/NM100A_Motor Velocity Control Function Requirement)' '#NM100A_49' 'true' 'REQ:  NM100A_49' '' ; 'linktype_rmi_doors' '00010020 (/E-STEER Core/SubSystem Specifications/Manufacturing Service/NM100A_Motor Velocity Control Function Requirement)' '#NM100A_51' 'true' 'REQ:  NM100A_51' '' ; 'linktype_rmi_doors' '00010020 (/E-STEER Core/SubSystem Specifications/Manufacturing Service/NM100A_Motor Velocity Control Function Requirement)' '#NM100A_103' 'true' 'REQ:  NM100A_103' '' ; 'linktype_rmi_doors' '00010020 (/E-STEER Core/SubSystem Specifications/Manufacturing Service/NM100A_Motor Velocity Control Function Requirement)' '#NM100A_130' 'true' 'REQ:  NM100A_130' '' } %GIDa_214f0c17_e692_4fb0_8ef6_fb165d366702"  NumInputs=4  IfExpression=u1  ElseIfExpressions=u2, ~u3, u4
  Mux : Mux  Inputs=9
  SlewMotVelTar : Subsystem
  State 1 : Subsystem  RequirementInfo={} %GIDa_8c6205ae_5932_444d_8028_d45b85e6549f  TreatAsAtomicUnit=on
  State 2 : Subsystem  RequirementInfo={} %GIDa_facb0b74_d7f2_406b_9dad_c80376ac3792  TreatAsAtomicUnit=on
  State 3 : Subsystem  TreatAsAtomicUnit=on
  State 4 : Subsystem  TreatAsAtomicUnit=on
  State 5 Do Nothing : Subsystem  RequirementInfo="{'linktype_rmi_doors' '00010020 (/E-STEER Core/SubSystem Specifications/Manufacturing Service/NM100A_Motor Velocity Control Function Requirement)' '#NM100A_130' 'true' 'REQ:  NM100A_130' '' } %GIDa_98eb7df3_8694_41df_8447_cf3eafeb5855"  TreatAsAtomicUnit=on
  wires:
  MotVelCrf/1 -> Mux/2
  SlewMotVelTar/1(MotVelTarSlewed) -> [MotVelTarSlewed]
  Data Store Read/1 -> If/1
  Data Store Read1/1 -> If/2
  Data Store Read2/1 -> If/3
  Data Store Read3/1 -> If/4
  If/1 -> State 1/Action
  [InpSig] -> State 1/1("InpSig ")
  If/2 -> State 2/Action
  [InpSig] -> State 2/1("InpSig ")
  If/3 -> State 3/Action
  If/4 -> State 4/Action
  If/5 -> State 5 Do Nothing/Action
  [MotVelTarSlewed] -> Mux/1
  PropGain/1 -> Mux/3
  IntgtrGain/1 -> Mux/4
  DerivtvGain/1 -> Mux/5
  AntiWdupLim/1 -> Mux/7
  AntiWdupGain/1 -> Mux/6
  DerivtvLpFilTiCon/1 -> Mux/8
  TqCmdLim/1 -> Mux/9
  Mux/1 -> [InpSig]
  [InpSig] -> State 3/1("InpSig ")

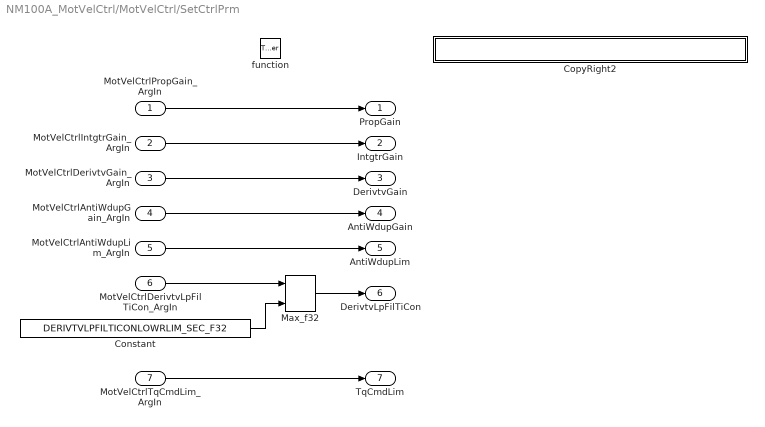
== system NM100A_MotVelCtrl/MotVelCtrl/SetCtrlPrm ==
  MotVelCtrlPropGain_ArgIn : Inport
  MotVelCtrlIntgtrGain_ArgIn : Inport  Port=2
  MotVelCtrlDerivtvGain_ArgIn : Inport  Port=3
  MotVelCtrlAntiWdupGain_ArgIn : Inport  Port=4
  MotVelCtrlAntiWdupLim_ArgIn : Inport  Port=5
  MotVelCtrlDerivtvLpFilTiCon_ArgIn : Inport  Port=6
  MotVelCtrlTqCmdLim_ArgIn : Inport  Port=7
  function : TriggerPort  TriggerType=function-call
  Constant : Constant  Value=DERIVTVLPFILTICONLOWRLIM_SEC_F32
  CopyRight2 : Subsystem  Description=|  mask(Copyright Information){none=on}
      | Copyright info block.                                               
      |                                                                     
      | Place copyright information at the top of every subsystem in design.
      mask prompts: none "No parameters"
      mask help: Place copyright information at the top of every subsystem in design.
      mask Display:
      | NxtrConf = 'Nexteer Confidential';
      | 
      | sys = bdroot; %handle for the current model ("system")
      | first = get_param(sys,'Created');
      | if(isempty(first))
      |     first = datestr(now,'yyyy');
      | else
      |     first = first(end-3:end);  %year is last four digits
      | end
      | 
      | last = get_param(sys,'LastModifiedDate');
      | if isempty(last)
      |     last = datestr(now,'yyyy');
      | else
      |     last = last(end-3:end);
      | end
      | 
      | if strcmp(first,last)
      |     fprintf('%s -- Copyright %s Nexteer',NxtrConf,first)
      | else
      |     fprintf('%s -- %s%s- %s Nexteer',NxtrConf,char(169),first,last)
      | end
  Max_f32 : NxtrMax/Max_f32  SFunctionSpec=single y1 = Max_f32(single u1, single u2)
      settings: AttributesFormatString=%<Name>
  PropGain : Outport
  IntgtrGain : Outport  Port=2
  DerivtvGain : Outport  Port=3
  AntiWdupGain : Outport  Port=4
  AntiWdupLim : Outport  Port=5
  DerivtvLpFilTiCon : Outport  Port=6
  TqCmdLim : Outport  Port=7
  wires:
  MotVelCtrlPropGain_ArgIn/1 -> PropGain/1
  MotVelCtrlIntgtrGain_ArgIn/1 -> IntgtrGain/1
  MotVelCtrlDerivtvGain_ArgIn/1 -> DerivtvGain/1
  MotVelCtrlAntiWdupGain_ArgIn/1 -> AntiWdupGain/1
  MotVelCtrlAntiWdupLim_ArgIn/1 -> AntiWdupLim/1
  MotVelCtrlDerivtvLpFilTiCon_ArgIn/1 -> Max_f32/1
  MotVelCtrlTqCmdLim_ArgIn/1 -> TqCmdLim/1
  Max_f32/1 -> DerivtvLpFilTiCon/1
  Constant/1 -> Max_f32/2

== system NM100A_MotVelCtrl/MotVelCtrl/StopCtrl ==
  MotVelCtrlVelSlewRate_ArgIn : Inport
  function : TriggerPort  TriggerType=function-call
  Constant : Constant  RequirementInfo={} %GIDa_0d3e0dec_2793_4810_8a92_94440cb47924  Value=ZEROMOTVELTAR_MOTRADPERSEC_F32
  Constant1 : Constant  RequirementInfo="{'linktype_rmi_doors' '00010020 (/E-STEER Core/SubSystem Specifications/Manufacturing Service/NM100A_Motor Velocity Control Function Requirement)' '#NM100A_87' 'true' 'REQ:  NM100A_87' '' } %GIDa_7618f473_7b18_4797_9c5d_069083555eac"  Value=FALSE_CNT_LGC
  CopyRight2 : Subsystem  Description=|  mask(Copyright Information){none=on}
      | Copyright info block.                                               
      |                                                                     
      | Place copyright information at the top of every subsystem in design.
      mask prompts: none "No parameters"
      mask help: Place copyright information at the top of every subsystem in design.
      mask Display:
      | NxtrConf = 'Nexteer Confidential';
      | 
      | sys = bdroot; %handle for the current model ("system")
      | first = get_param(sys,'Created');
      | if(isempty(first))
      |     first = datestr(now,'yyyy');
      | else
      |     first = first(end-3:end);  %year is last four digits
      | end
      | 
      | last = get_param(sys,'LastModifiedDate');
      | if isempty(last)
      |     last = datestr(now,'yyyy');
      | else
      |     last = last(end-3:end);
      | end
      | 
      | if strcmp(first,last)
      |     fprintf('%s -- Copyright %s Nexteer',NxtrConf,first)
      | else
      |     fprintf('%s -- %s%s- %s Nexteer',NxtrConf,char(169),first,last)
      | end
  Data Store Write : DataStoreWrite  RequirementInfo={} %GIDa_2102ddea_8f05_4652_878d_08a25dab01f4  DataStoreName=MotVelTar
  Data Store Write1 : DataStoreWrite  DataStoreName=VelSlewRate
  Data Store Write2 : DataStoreWrite  RequirementInfo="{'linktype_rmi_doors' '00010020 (/E-STEER Core/SubSystem Specifications/Manufacturing Service/NM100A_Motor Velocity Control Function Requirement)' '#NM100A_87' 'true' 'REQ:  NM100A_87' '' } %GIDa_86970bdf_df91_4611_b5e7_f17f8c3f6f1e"  DataStoreName=EnaCtrl
  wires:
  Constant/1 -> Data Store Write/1
  MotVelCtrlVelSlewRate_ArgIn/1 -> Data Store Write1/1
  Constant1/1 -> Data Store Write2/1

== system NM100A_MotVelCtrl/MotVelCtrl/StrtCtrl ==
  MotVelCtrlMotVelTar_ArgIn : Inport  RequirementInfo={} %GIDa_a4226ff9_0a68_4d3b_91a4_7e41e7c74922
  MotVelCtrlVelSlewRate_ArgIn : Inport  RequirementInfo={} %GIDa_906ab9ae_6c20_455d_8452_d169d695b146  Port=2
  function : TriggerPort  TriggerType=function-call
  Constant : Constant  RequirementInfo="{'linktype_rmi_doors' '00010020 (/E-STEER Core/SubSystem Specifications/Manufacturing Service/NM100A_Motor Velocity Control Function Requirement)' '#NM100A_93' 'true' 'REQ:  NM100A_93' '' } %GIDa_f2e6fa93_2156_4235_82a1_0a95b9a77abc"  Value=TRUE_CNT_LGC
  CopyRight2 : Subsystem  Description=|  mask(Copyright Information){none=on}
      | Copyright info block.                                               
      |                                                                     
      | Place copyright information at the top of every subsystem in design.
      mask prompts: none "No parameters"
      mask help: Place copyright information at the top of every subsystem in design.
      mask Display:
      | NxtrConf = 'Nexteer Confidential';
      | 
      | sys = bdroot; %handle for the current model ("system")
      | first = get_param(sys,'Created');
      | if(isempty(first))
      |     first = datestr(now,'yyyy');
      | else
      |     first = first(end-3:end);  %year is last four digits
      | end
      | 
      | last = get_param(sys,'LastModifiedDate');
      | if isempty(last)
      |     last = datestr(now,'yyyy');
      | else
      |     last = last(end-3:end);
      | end
      | 
      | if strcmp(first,last)
      |     fprintf('%s -- Copyright %s Nexteer',NxtrConf,first)
      | else
      |     fprintf('%s -- %s%s- %s Nexteer',NxtrConf,char(169),first,last)
      | end
  Data Store Write : DataStoreWrite  RequirementInfo={} %GIDa_991f57cc_b740_4c25_b84a_977fef87c7de  DataStoreName=MotVelTar
  Data Store Write1 : DataStoreWrite  RequirementInfo={} %GIDa_42433dbb_b1b7_474b_a7ce_c257b55188f2  DataStoreName=VelSlewRate
  Data Store Write2 : DataStoreWrite  RequirementInfo="{'linktype_rmi_doors' '00010020 (/E-STEER Core/SubSystem Specifications/Manufacturing Service/NM100A_Motor Velocity Control Function Requirement)' '#NM100A_93' 'true' 'REQ:  NM100A_93' '' } %GIDa_2a7f9af6_b8e8_4d99_85ec_d5b5cf9e2d93"  DataStoreName=EnaCtrl
  wires:
  MotVelCtrlMotVelTar_ArgIn/1 -> Data Store Write/1
  MotVelCtrlVelSlewRate_ArgIn/1 -> Data Store Write1/1
  Constant/1 -> Data Store Write2/1

== system NM100A_MotVelCtrl/MotVelCtrl/GetCtrlPrm/CopyRight2 ==

== system NM100A_MotVelCtrl/MotVelCtrl/MotVelCtrlInit1/CopyRight2 ==

== system NM100A_MotVelCtrl/MotVelCtrl/MotVelCtrlPer1/CopyRight2 ==

== system NM100A_MotVelCtrl/MotVelCtrl/MotVelCtrlPer1/SlewMotVelTar ==
  CopyRight2 : Subsystem  Description=|  mask(Copyright Information){none=on}
      | Copyright info block.                                               
      |                                                                     
      | Place copyright information at the top of every subsystem in design.
      mask prompts: none "No parameters"
      mask help: Place copyright information at the top of every subsystem in design.
      mask Display:
      | NxtrConf = 'Nexteer Confidential';
      | 
      | sys = bdroot; %handle for the current model ("system")
      | first = get_param(sys,'Created');
      | if(isempty(first))
      |     first = datestr(now,'yyyy');
      | else
      |     first = first(end-3:end);  %year is last four digits
      | end
      | 
      | last = get_param(sys,'LastModifiedDate');
      | if isempty(last)
      |     last = datestr(now,'yyyy');
      | else
      |     last = last(end-3:end);
      | end
      | 
      | if strcmp(first,last)
      |     fprintf('%s -- Copyright %s Nexteer',NxtrConf,first)
      | else
      |     fprintf('%s -- %s%s- %s Nexteer',NxtrConf,char(169),first,last)
      | end
  Data Store Read : DataStoreRead  RequirementInfo="{'linktype_rmi_doors' '00010020 (/E-STEER Core/SubSystem Specifications/Manufacturing Service/NM100A_Motor Velocity Control Function Requirement)' '#NM100A_28' 'true' 'REQ:  NM100A_28' '' } %GIDa_4b650935_bde1_4022_8cb0_1ea9b415e9d2"  DataStoreName=MotVelTar
  Data Store Read1 : DataStoreRead  RequirementInfo="{'linktype_rmi_doors' '00010020 (/E-STEER Core/SubSystem Specifications/Manufacturing Service/NM100A_Motor Velocity Control Function Requirement)' '#NM100A_28' 'true' 'REQ:  NM100A_28' '' } %GIDa_56abd541_633e_43e8_9638_eb268ad61042"  DataStoreName=VelSlewRate
  RateLimDyn_f32 : NxtrLim/RateLimDyn_f32  RequirementInfo="{'linktype_rmi_doors' '00010020 (/E-STEER Core/SubSystem Specifications/Manufacturing Service/NM100A_Motor Velocity Control Function Requirement)' '#NM100A_28' 'true' 'REQ:  NM100A_28' '' } %GIDa_4fb99026_3798_453c_9a26_a13ec02574ad"  StVar=PrevMotVelTar  Ts=ARCHGLBPRM_2MILLISEC_SEC_F32
      settings: AttributesFormatString=StVar: %<StVar>
  Unary Minus : UnaryMinus  RequirementInfo="{'linktype_rmi_doors' '00010020 (/E-STEER Core/SubSystem Specifications/Manufacturing Service/NM100A_Motor Velocity Control Function Requirement)' '#NM100A_28' 'true' 'REQ:  NM100A_28' '' } %GIDa_7d612f8c_1237_4dfa_8652_dd4d7a6abcc2"
  MotVelTarSlewed : Outport  RequirementInfo="{'linktype_rmi_doors' '00010020 (/E-STEER Core/SubSystem Specifications/Manufacturing Service/NM100A_Motor Velocity Control Function Requirement)' '#NM100A_28' 'true' 'REQ:  NM100A_28' '' } %GIDa_6fa68041_9688_4ded_8328_e5865332680e"
  wires:
  Data Store Read/1 -> RateLimDyn_f32/1
  Unary Minus/1 -> RateLimDyn_f32/2
  RateLimDyn_f32/1 -> MotVelTarSlewed/1
  Data Store Read1/1 -> RateLimDyn_f32/3, Unary Minus/1

== system NM100A_MotVelCtrl/MotVelCtrl/MotVelCtrlPer1/State 1 ==
  note: Client call SetManTqCmd in SF04 AssiSumLim
  "InpSig " : Inport
  Action Port : ActionPort  ActionType=then
  Constant : Constant  RequirementInfo="{'linktype_rmi_doors' '00010020 (/E-STEER Core/SubSystem Specifications/Manufacturing Service/NM100A_Motor Velocity Control Function Requirement)' '#NM100A_48' 'true' 'REQ:  NM100A_48' '' } %GIDa_606f8acf_aecb_49cf_a2fb_b318bb4ec03f"  Value=TRUE_CNT_LGC
  Constant1 : Constant  RequirementInfo="{'linktype_rmi_doors' '00010020 (/E-STEER Core/SubSystem Specifications/Manufacturing Service/NM100A_Motor Velocity Control Function Requirement)' '#NM100A_48' 'true' 'REQ:  NM100A_48' '' } %GIDa_252597c8_55b3_4b7f_a33d_e916075b511b"  Value=TRUE_CNT_LGC
  CopyRight2 : Subsystem  Description=|  mask(Copyright Information){none=on}
      | Copyright info block.                                               
      |                                                                     
      | Place copyright information at the top of every subsystem in design.
      mask prompts: none "No parameters"
      mask help: Place copyright information at the top of every subsystem in design.
      mask Display:
      | NxtrConf = 'Nexteer Confidential';
      | 
      | sys = bdroot; %handle for the current model ("system")
      | first = get_param(sys,'Created');
      | if(isempty(first))
      |     first = datestr(now,'yyyy');
      | else
      |     first = first(end-3:end);  %year is last four digits
      | end
      | 
      | last = get_param(sys,'LastModifiedDate');
      | if isempty(last)
      |     last = datestr(now,'yyyy');
      | else
      |     last = last(end-3:end);
      | end
      | 
      | if strcmp(first,last)
      |     fprintf('%s -- Copyright %s Nexteer',NxtrConf,first)
      | else
      |     fprintf('%s -- %s%s- %s Nexteer',NxtrConf,char(169),first,last)
      | end
  Data Store Read : DataStoreRead  RequirementInfo={} %GIDa_a431b5c4_f353_4542_b98c_225abc5d2410  DataStoreName=EnaCtrl
  Data Store Write : DataStoreWrite  RequirementInfo="{'linktype_rmi_doors' '00010020 (/E-STEER Core/SubSystem Specifications/Manufacturing Service/NM100A_Motor Velocity Control Function Requirement)' '#NM100A_48' 'true' 'REQ:  NM100A_48' '' } %GIDa_588e0a52_df3e_4d53_a996_cc6f3362f8b8"  DataStoreName=FctActvSts
  Data Store Write1 : DataStoreWrite  RequirementInfo={} %GIDa_7e07712d_915c_4cca_808e_f9ea5cc32bee  DataStoreName=EnaCtrlStVari
  Demux : Demux  Outputs=9
  F_PID Control_1 : Subsystem
  SetManTqCmd : Subsystem  RequirementInfo={} %GIDa_78939431_2206_43a1_80f2_271873b982fd
  wires:
  Constant/1 -> Data Store Write/1
  Data Store Read/1 -> Data Store Write1/1
  Constant1/1 -> SetManTqCmd/2(ManTqCmdEna)
  F_PID Control_1/1("PIDCmd ") -> [PIDCmd]
  [PIDCmd] -> SetManTqCmd/1(ManTqCmd)
  "InpSig "/1 -> Demux/1
  Demux/9 -> F_PID Control_1/9(TqCmdLim)
  Demux/8 -> F_PID Control_1/8(DerivtvLpFilTiCon)
  Demux/1 -> F_PID Control_1/1(MotVelTarSlewed)
  Demux/2 -> F_PID Control_1/2(MotVelCrf)
  Demux/3 -> F_PID Control_1/3(PropGain)
  Demux/4 -> F_PID Control_1/4(IntgtrGain)
  Demux/5 -> F_PID Control_1/5(DerivtvGain)
  Demux/6 -> F_PID Control_1/6(AntiWdupGain)
  Demux/7 -> F_PID Control_1/7(AntiWdupLim)
